simulink model "BiT_Template_V4"  (R2025b)
settings: Solver=FixedStepAuto  StartTime=0.0  StopTime=90  FixedStep=0.005  RelTol=1e-3
StopFcn:
  | user_confirmed = true;
  | disp('Gestoppt?!')
  | 
  | % stop(t);
  | % delete(t);
  | 
  | %% Switch to Config Mode
  | %Tc3_AI.sysManager.ActivateConfiguration();
  | %
  | % Tc3_AI.SwitchToConfig('local')
  | %
  | % %save Solution
  | % Tc3_AI.SaveSolution();
  | %
  | % %% Close Aktive VS Instance
  | % Tc3_AI.closeVsInstance();
libraries: simulink x1, slpidlib x1
settings Model: SimulationMode=external  Creator=clemensm  LastModifiedBy=Felix
settings OptimizationCC: LocalBlockOutputs=off
settings RTWCC: SystemTargetFile=TwinCatGrt.tlc  GenCodeOnly=on  GenerateMakefile=off  TemplateMakefile=tcgrt_msbuild.tmf  TargetLang=C++  Description=TwinCAT GRT Target
settings STFCustomTargetCC: SystemTargetFile=TwinCatGrt.tlc  TargetLangStandard=C++11 (ISO)  CombineOutputUpdateFcns=on  CodeInterfacePackaging=Reusable function  CPPClassGenCompliant=on  GRTInterface=off  GenerateAllocFcn=on  TcProject_PublishPlatformtoolset=Auto  TcCom_DWorkCreateSymbols=on  TcCom_UpdateExceptionHandling=CallerExceptions  TcCom_OriginalIoBlockNames=off  TcProject_UseCodeDescriptor=on  TcCom_ContStateDataAccess=Internal DataArea  TcCom_StepSizeAdaptation=RequireMatchingTaskCycleTime  TcProject_InstallPlcLibrary=off  TcCom_OutputReadOnly=on  TcCom_ModuleIcon=$<TE140x:Icon>  TcProject_LibraryCategories=$<VendorName>  TcProject_SignTwinCatCertName=MCI_2024_OEM.tccert  TcCom_ResolveMaskedSubsystems=on  TcProject_PublishParallel=on  TcCom_StrictAccessLock=on  TcProject_TmxInstall=on  TcPlcFb_Generate=off  TcCom_ExecutionInfoParam=on  TcProject_Generate=on  TcCom_ExtModeRtAllowForParameterChange=on  TcCom_OutputDataAccess=Output Source DataArea  TcCom_DWorkReadOnly=on  TcCom_ParametersDataAccess=Internal DataArea  TcCom_DataStoreCreateSymbols=on  TcCom_InputReadOnly=off  TcCom_BlockIoDataAccess=Internal DataArea  TcProject_IncrementVersion=Revision  TcProject_CoderCppNamespace=coder  TcCom_DWorkDataAccess=Internal DataArea  TcProject_UseCodeInfoExporter=on  TcProject_LibCatPath=$<Project:Dir>\$<Project:Name>.libcat.xml  TcCom_GlobalParamDefaultSharing=Define  TcCom_ExecutionInfoOutput=off  TcProject_PublishTcRTx64=on  TcCom_OutputCreateSymbols=on  TcProject_Copyright=Copyright $<VendorName> $<LocalDateTime:%Y>  TcProject_DataExchangeModulesVersion=$<ModuleGenerator:DataExchange:Version>  TcCom_ExtendSignalResolution=on  TcProject_ProductName=$<ModuleGenerator:ProductId> $<ModuleGenerator:Version:MAJOR.MINOR>  TcProject_PreferToolArchitectureX64=on  TcProject_DeployRestart=off  TcCom_GroupName=TE140x|Simulink Modules  TcProject_PlcVarPrefixes=PVOID=p | BOOL=b | BOOL32=b | DATE=d | TIME_OF_DATE=td | TIME=t | LTIME=t | GUID=n  TcCom_TcComWrapperFbProperties=off  TcProject_LowestCompatibleTcBuild=$<TwinCAT:Version:BUILD>  TcProject_PublishTcOSARMv7A=off  TcProject_GenerateVsSolution=No  TcProject_Description=TwinCAT executable file, generated by TwinCAT $<ModuleGenerator:ProductId>  TcProject_CreateScopedEnums=Auto  TcCom_GroupDisplayName=$<GroupName>  TcCom_InputCreateSymbols=on  TcProject_PublishTcOSx64=off  TcCom_OnlineChange=off  TcCom_ModuleCaller=CyclicTask  TcCom_ExecutionSequence=UpdateBeforeOutputMapping  TcPlcFb_InitExceptionHandling=CallerExceptions  TcCom_AllowDataAreaForSharedData=off  TcPlcFb_OemLicenses=$<Project:OemLicenses>  TcCom_InitExceptionHandling=CallerExceptions  TcCom_DataStoreDataAccess=None  TcCom_AccessLockState=Auto  TcCom_BlockDiagramDebugInfoExport=on  TcCom_ContStateCreateSymbols=on  TcCom_Legacy_ModuleBuildInfoParam=on  TcCom_MonitorExecutionTime=off  TcProject_ProjectDir=C:\TwinCAT\3.1\CustomConfig\Modules\Ctrl_only  TcCom_InputDataAccess=Input Destination DataArea  TcCom_BlockDiagramExport=on  TcCom_ExecuteModelCode=on  TcPlcFb_MonitorExecutionTime=off  TcPlcFb_ExtModeRtAllowForParameterChange=off  TcCom_ExtModeRtWaitForStart=off  TcProject_PublishTcOSARMv8A=off  TcProject_VendorName=TE140x Module Vendor  TcProject_GenerateStructDutsWithDefaultValues=Auto  TcCom_CallerVerification=Default  TcProject_ClassFactoryName=$<Project:Name>  TcCom_InputInitValues=off  TcProject_DrvProductVersion=$<DrvFileVersion>  TcProject_PreferIntOverLong=off  TcCom_OemLicenses=$<Project:OemLicenses>  TcPlcFb_ExtModeRtWaitForStart=off  TcCom_TcComWrapperFb=off  TcCom_GroupIcon=$<TE140x:Icon>  TcProject_UseTmxExtension=Auto  TcProject_CppLanguageStandard=Default  TcCom_BlockIoReadOnly=on  TcProject_CreateUniqueEnumItemNames=off  TcPlcFb_ExtModeRtAllowExecutionCommands=off  TcProject_StaticStlStringCapacity=Auto  TcProject_DrvFileVersion=$<VersionFromFile>  TcProject_ForceRebuildForPublish=off  TcCom_BlockIoCreateSymbols=on  TcProject_SignWithTwinCatCertificate=inherit default  TcProject_UseNativeBlockDiagramExport=off  TcProject_GeneratePlcLibrary=off  TcProject_PublishTcOSARMv7M=off  TcCom_BlockDiagramVariableAccess=AssignToParent  TcProject_UseDataExchangeModules=off  TcProject_UseIntrinsics=on  TcProject_PublishTcRTx86=on  TcCom_ContStateReadOnly=on  TcCom_ParametersReadOnly=off  TcCom_Generate=on  TcCom_DataStoreReadOnly=off  TcProject_VendorIcon=$<TE140x:Icon>  TcProject_Versioning=Versioned  TcProject_Publish=on  TcProject_EnableNewPlatforms=off  TcProject_Verbosity=Normal  TcProject_UseStaticStlString=off  TcProject_CLanguageStandard=Default  TcProject_VersionSrc=$<LatestTMFile>  TcProject_BuildWithWdk=inherit default  TcProject_UseDescriptorCodeType=on  TcCom_ParametersInitValues=on  TcCom_TcComWrapperFbPropertyMonitoring=NoMonitoring  TcCom_VariableSymbolMapping=Identical  TcProject_PublishTcUMx86=off  TcProject_BuildSystem=Auto  TcPlcFb_UpdateExceptionHandling=CallerExceptions  TcProject_PublishTcUMx64=off  TcProject_PublishConfiguration=Release  TcCom_ExtModeRtAllowExecutionCommands=on  TcCom_ParametersCreateSymbols=on  TcProject_MaxVisibleArrayElements=200U  TcCom_OnlineChangeRestoreDataAreas=off
settings GRTTargetCC: ExtMode=on  ExtModeMexFile=TcExtModeClient  MultiInstanceErrorCode=None  TargetLangStandard=C++11 (ISO)  ParMdlRefBuildCompliant=off  CompOptLevelCompliant=off  MatFileLogging=off  CodeInterfacePackaging=Reusable function  GenerateAllocFcn=on  UseToolchainInfoCompliant=off

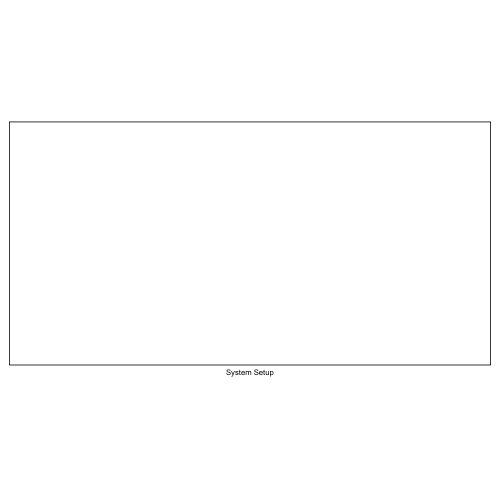
[thumbnail: Simulink's stored preview of the top-level diagram]
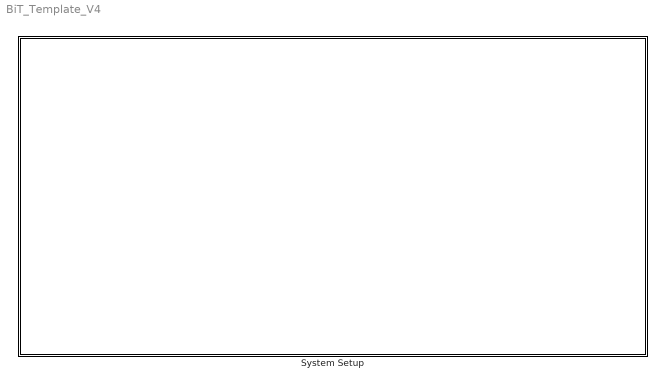
== system BiT_Template_V4 ==
  System Setup : Subsystem

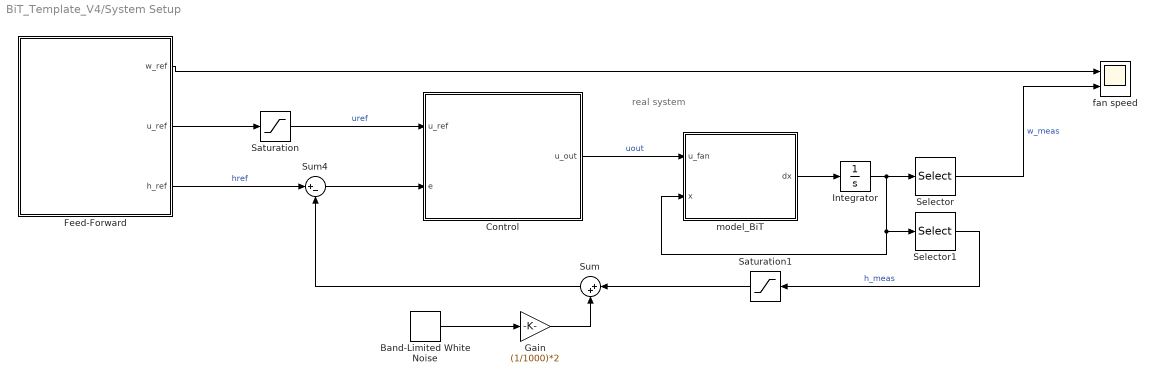
== system BiT_Template_V4/System Setup ==
  note: real system
  Band-Limited White Noise : simulink/Sources/Band-Limited White Noise  Cov=[0.9]  Ts=0.1  seed=[23341]
  Control : Subsystem
  Feed-Forward : Subsystem
  Gain : Gain  Gain=(1/1000)*2
  Integrator : Integrator  InitialCondition=[0.1;0;4200]  UpperSaturationLimit=[0.5;5;8000]  LowerSaturationLimit=0
  Saturation : Saturate  UpperLimit=100  LowerLimit=0
  Saturation1 : Saturate  LowerLimit=0
  Selector : Selector  InputPortWidth=3  IndexOptions=Index vector (dialog)  Indices=3  OutputSizes=1
  Selector1 : Selector  InputPortWidth=3  IndexOptions=Index vector (dialog)  Indices=1  OutputSizes=1
  Sum : Sum  Inputs=|++
  Sum4 : Sum  Inputs=|+-
  fan speed : Scope  NumInputPorts=2
      settings: TimeSpan=60  ActiveDisplayYMinimum=4192.4462547686062  ActiveDisplayYMaximum=4423.0615272479326
  model_BiT : MATLAB Function  TreatAsAtomicUnit=on
  wires:
  Selector/1 -> fan speed/2  "w_meas"
  Integrator/1 -> Selector/1, Selector1/1, model_BiT/2(x)
  Feed-Forward/1(w_ref) -> fan speed/1
  Sum4/1 -> Control/2(e)
  Feed-Forward/2(u_ref) -> Saturation/1
  Feed-Forward/3(h_ref) -> Sum4/1  "href"
  Saturation/1 -> Control/1(u_ref)  "uref"
  Band-Limited White Noise/1 -> Gain/1
  Control/1(u_out) -> model_BiT/1(u_fan)  "uout"
  model_BiT/1(dx) -> Integrator/1
  Selector1/1 -> Saturation1/1  "h_meas"
  Sum/1 -> Sum4/2
  Gain/1 -> Sum/2
  Saturation1/1 -> Sum/1

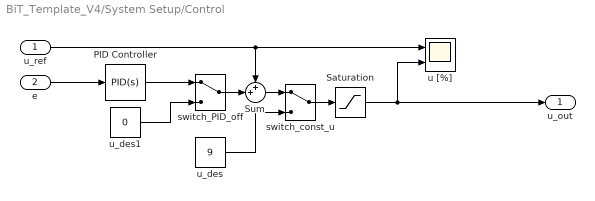
== system BiT_Template_V4/System Setup/Control ==
  u_ref : Inport
  e : Inport  Port=2
  PID Controller : slpidlib/PID Controller  Controller=PID  Form=Parallel  TimeDomain=Continuous-time  UseExternalTs=off  SampleTime=-1  IntegratorMethod=Forward Euler  FilterMethod=Forward Euler  ControllerParametersSource=internal  P=1  I=0.1  UseKiTs=off  D=1  UseExternalDerivativeSource=off  N=100  UseFilter=on  TunerSelectOption=Transfer Function Based (PID Tuner App)  InitialConditionSource=internal  InitialConditionForIntegrator=0  InitialConditionForFilter=0  DifferentiatorICPrevScaledInput=0  ExternalReset=none  TrackingMode=off  Kt=1  LimitOutput=off  SatLimitsSource=internal  UpperSaturationLimit=inf  LowerSaturationLimit=-inf  LinearizeAsGain=on  AntiWindupMode=none  Kb=1  LimitIntegrator=off  UpperIntegratorSaturationLimit=inf  LowerIntegratorSaturationLimit=-inf  POutMin=[]  POutMax=[]  IOutMin=[]  IOutMax=[]  DOutMin=[]  DOutMax=[]  NOutMin=[]  NOutMax=[]  SumOutMin=[]  SumOutMax=[]  SaturationOutMin=[]  SaturationOutMax=[]  PParamMin=[]  PParamMax=[]  IParamMin=[]  IParamMax=[]  DParamMin=[]  DParamMax=[]  NParamMin=[]  NParamMax=[]  KbParamMin=[]  KbParamMax=[]  KtParamMin=[]  KtParamMax=[]  KbOutMin=[]  KbOutMax=[]  KtOutMin=[]  KtOutMax=[]  IntegratorOutMin=[]  IntegratorOutMax=[]  FilterOutMin=[]  FilterOutMax=[]  SumI1OutMin=[]  SumI1OutMax=[]  SumI2OutMin=[]  SumI2OutMax=[]  SumI3OutMin=[]  SumI3OutMax=[]  SumI4OutMin=[]  SumI4OutMax=[]  SumDOutMin=[]  SumDOutMax=[]  DifferentiatorOutMin=[]  DifferentiatorOutMax=[]  FilterDiffOutCoefMin=[]  FilterDiffOutCoefMax=[]  ReciprocalOutMin=[]  ReciprocalOutMax=[]  SumDenOutMin=[]  SumDenOutMax=[]  SumNumOutMin=[]  SumNumOutMax=[]  DivideOutMin=[]  DivideOutMax=[]  UdiffTsProdOutMin=[]  UdiffTsProdOutMax=[]  NTsProdOutMin=[]  NTsProdOutMax=[]  UintegralTsProdOutMin=[]  UintegralTsProdOutMax=[]  UngainTsProdOutMin=[]  UngainTsProdOutMax=[]  ClampingZeroOutDataTypeStr=Inherit: Inherit via back propagation  ClampingZeroOutMin=[]  ClampingZeroOutMax=[]  FilterDenConstantOutDataTypeStr=Inherit: Inherit via back propagation  FilterDenConstantOutMin=[]  FilterDenConstantOutMax=[]  PCopyOutDataTypeStr=Inherit: Inherit via back propagation  PCopyOutMin=[]  PCopyOutMax=[]  NCopyOutDataTypeStr=Inherit: Inherit via back propagation  NCopyOutMin=[]  NCopyOutMax=[]  IntegratorContinuousStateAttributes=''  IntegratorStateMustResolveToSignalObject=off  IntegratorRTWStateStorageClass=Auto  FilterContinuousStateAttributes=''  FilterStateMustResolveToSignalObject=off  FilterRTWStateStorageClass=Auto  ParallelPVariant=InternalParameters  IdealPVariant=Disabled  IVariant=InternalParameters  DVariant=InternalParameters  IntegratorVariant=Continuous  SatVariant=Disabled  AWVariant=Passthrough  PCopyVariant=Disabled  TRVariant=Disabled  FdbkBlocksVariant=Forward  IdealPFdbkVariant=Disabled  SatFdbkVariant=Disabled  DerivativeFilterVariant=ContFilter  NVariant=InternalParameters  NCopyVariant=Disabled  FilterICVariant=InternalICsFilter  IntegratorICVariant=InternalICs  ExternalResetVariant=Disabled  TRSumVariant=Passthrough  SumFdbkVariant=Disabled  SumVariant=Sum_PID  TsampFilterVariant=InternalTs  TsampNgainVariant=Passthrough  TsampIntegralVariant=Disabled_SignalSpec  ExternalSaturationOutDataTypeStr=Inherit: Same as second input  DerivativeSourceVariant=ErrorSignal  PreIntVariant=InternalPreInt
  Saturation : Saturate  UpperLimit=100  LowerLimit=0
  Sum : Sum  Inputs=++|
  switch_PID_off : ManualSwitch
  switch_const_u : ManualSwitch
  u [%] : Scope  NumInputPorts=2
      settings: TimeSpan=60  ActiveDisplayYMinimum=7.1623782098242694  ActiveDisplayYMaximum=10.402299316136082
  u_des : Constant  Value=9
  u_des1 : Constant  Value=0
  u_out : Outport
  wires:
  e/1 -> PID Controller/1
  u_ref/1 -> u [%]/1, Sum/1
  Sum/1 -> switch_const_u/1
  PID Controller/1 -> switch_PID_off/1
  switch_PID_off/1 -> Sum/2
  u_des1/1 -> switch_PID_off/2
  Saturation/1 -> u_out/1, u [%]/2
  switch_const_u/1 -> Saturation/1
  u_des/1 -> switch_const_u/2

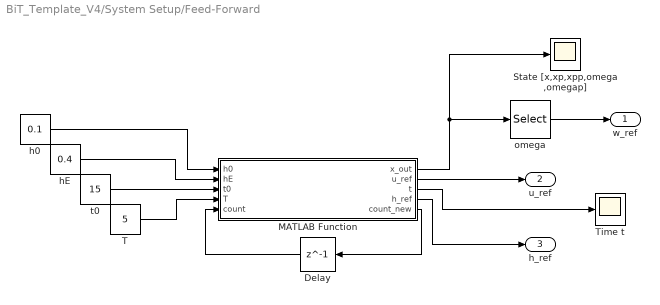
== system BiT_Template_V4/System Setup/Feed-Forward ==
  Delay : Delay  DelayLength=1
  MATLAB Function : MATLAB Function  TreatAsAtomicUnit=on
  State [x,xp,xpp,omega,omegap] : Scope
      settings: TimeSpan=60  ActiveDisplayYMinimum=-2.8507281834226665  ActiveDisplayYMaximum=4.5348179296068727
  T : Constant  Value=5
  Time t : Scope
      settings: ActiveDisplayYMinimum=-1  ActiveDisplayYMaximum=1
  h0 : Constant  Value=0.1
  hE : Constant  Value=0.4
  omega : Selector  InputPortWidth=5  IndexOptions=Index vector (dialog)  Indices=4  OutputSizes=1
  t0 : Constant  Value=15
  w_ref : Outport
  u_ref : Outport  Port=2
  h_ref : Outport  Port=3
  wires:
  h0/1 -> MATLAB Function/1(h0)
  MATLAB Function/3(t) -> Time t/1
  T/1 -> MATLAB Function/4(T)
  t0/1 -> MATLAB Function/3(t0)
  Delay/1 -> MATLAB Function/5(count)
  MATLAB Function/5(count_new) -> Delay/1
  hE/1 -> MATLAB Function/2(hE)
  MATLAB Function/1(x_out) -> State [x,xp,xpp,omega,omegap]/1, omega/1
  MATLAB Function/2(u_ref) -> u_ref/1
  MATLAB Function/4(h_ref) -> h_ref/1
  omega/1 -> w_ref/1

== matlab function BiT_Template_V4/System Setup/model_BiT ==
  data: u_fan input; dx output; x input
function dx = model_BiT(u_fan, x)

alpha1 = 0.000745736;
alpha2 = 0.209195;
alpha3 = 9.81;
tau_omega = 1.255; 
u_0 = -34.234; 
k_omega = 96.295;

dx1 = x(2);
dx2 = (alpha1*x(3) - alpha2*x(2))^2 - alpha3;
dx3 = (k_omega*(u_fan-u_0)-x(3))/tau_omega;

dx = [dx1; dx2; dx3];
end

== matlab function BiT_Template_V4/System Setup/Feed-Forward/MATLAB Function ==
  data: x_out output; u_ref output; t output; h0 input; hE input; t0 input; T input; h_ref output; count input; count_new output
function [x_out,u_ref,t,h_ref,count_new] = feed_forward(h0,hE,t0,T,count)

count_new = count+1;
dT = 0.005;
t_total = count_new*dT;

n = floor(t_total/(t0 + T));
t = rem(t_total, (t0+T));

alpha1 = 0.000745736;
alpha2 = 0.209195;
alpha3 = 9.81;
tau_omega = 1.255; 
u_0 = -34.234; 
k_omega = 96.295;

xp_ref = 0;
xpp_ref = 0;
xppp_ref = 0;

if t<t0
    if rem(n, 2) == 0
        x_ref = h0;
    else
        x_ref = hE;
    end
elseif t>t0+T
    if rem(n, 2) == 0
        x_ref = hE;
    else
        x_ref = h0;
    end
else
    s = (t - t0)/T;
    x_ref = h0 - (h0 - hE) * (35*s.^4-84*s.^5 +70*s.^6 - 20*s.^7);
    xp_ref = -(h0 - hE) * (140*s.^3 - 420*s.^4 + 420*s.^5 - 140*s.^6) / T;
    xpp_ref = -(h0 - hE) * (420*s.^2 - 1680*s.^3 + 2100*s.^4 - 840*s.^5) / T^2;
    xppp_ref = -(h0 - hE) * (840*s - 5040*s.^2 + 8400*s.^3 - 4200*s.^4)/T^3;
end

acc = xpp_ref + alpha3;

omega = (sqrt(acc) + alpha2 * xp_ref) / alpha1;
omega_p = (xppp_ref/(2*sqrt(acc)) + alpha2*xpp_ref)/alpha1;

u = (tau_omega*omega_p + omega)/k_omega + u_0;

h_ref = x_ref;

u_min = 0;
u_max = 100;
u = max(min(u, u_max), u_min);

u_ref = u; 
x_out = [x_ref,xp_ref,xpp_ref,omega,omega_p]';
end
